simulink library "BodyLoad_Tank_Cylindrical"  (R2025b)
settings: Solver=VariableStepAuto  StartTime=0.0  StopTime=10.0  RelTol=1e-3
undefined symbols (not defined in the file): BodyLoad, X, Y, Z
libraries: sm_lib x4
Description:
  | Component of Simscape Vehicle Templates Library
  | 
  | Copyright 2018-2025 The MathWorks, Inc.
settings Model: Creator=smiller  LastModifiedBy=smiller
settings SolverCC: AlgebraicLoopSolver=TrustRegion
settings DataIOCC: ReturnWorkspaceOutputs=off
settings OptimizationCC: ReuseModelBlockBuffer=off
settings DebuggingCC: UnconnectedInputMsg=warning  UnconnectedOutputMsg=warning  UnconnectedLineMsg=warning  ArithmeticOperatorsInVariantConditions=warning
settings ModelReferenceCC: EnableRefExpFcnMdlSchedulingChecks=on
settings SFSimCC: CustomCodeUndefinedFunction=UseInterfaceOnly
settings RTWCC: GPUComputeCapability=3.5  DLArmComputeVersion=19.05

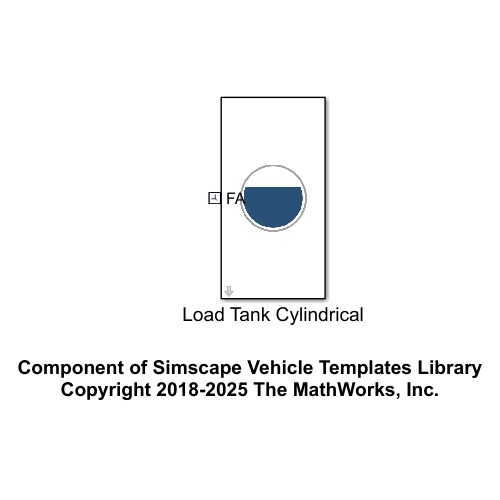
[thumbnail: Simulink's stored preview of the top-level diagram]
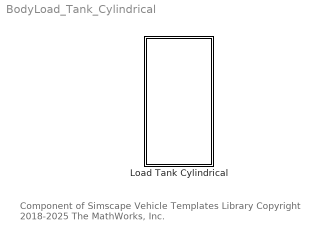
== system BodyLoad_Tank_Cylindrical ==
  note: Component of Simscape Vehicle Templates Library
      | Copyright 2018-2025 The MathWorks, Inc.
  Load Tank Cylindrical : Subsystem  mask(Inertial Load for Cylindrical Tank){refToTankCtr=BodyLoad.xRefToTankCtr.Value, tank_rad=BodyLoad.xRadius.Value, tank_len=BodyLoad.xLength.Value, pcnt_fill=BodyLoad.rFillHeight.Value, rho=BodyLoad.rho.Value, dLoad=BodyLoad.dLoad.Value, clr=BodyLoad.Color.Value, opc=BodyLoad.Opacity.Value}
      mask prompts: refToTankCtr "Ref to Tank Center [x y z] (m)"; tank_rad "Tank Radius (m)"; tank_len "Tank Length (m)"; pcnt_fill "Percent Fill Height (0-1)"; rho "Density (kg/m^3)"; dLoad "Load Rotational Damping (N*m/(deg/s))"; clr "Color [RGB]"; opc "Opacity (0-1)"
      mask help: Model the load in a full or partially full horizontal cylindrical tank subjected to gravity. Specify the size of the tank, density of the fluid, and how full the tank is. Tank fill level is specified as a percentage of the tank diameter. The load can slosh laterally by rotating around the tank axis. Slosh can be inibited by setting the Load Rotational Damping to a high value.
      mask init:
      | % Limit percent fill from 0-1
      | if(pcnt_fill>1)
      |     pcnt_fill = 1;
      | elseif(pcnt_fill<0)
      |     pcnt_fill = 0;
      | end
      | 
      | % Calculate angle for extrusion
      | if(pcnt_fill>0.5)
      |     fill_angle = pi/2+asin((pcnt_fill-0.5)*2);
      | else
      |     fill_angle = acos((0.5-pcnt_fill)*2);
      | end
      | 
      | % Create angle vector for extrusion
      | angle_vec = linspace(-fill_angle,fill_angle,50);
      | 
      | % Create extrusion data
      | xy_data_load = [(cos(angle_vec))' (sin(angle_vec))']*(tank_rad-1e-3);
      mask TypeOptions clr: Load/GraphicDiffuseColor
      mask TypeOptions opc: Load/GraphicOpacity
      mask DialogControl cont_vis Prompt: Visualization
      mask Display: image('sm_car_vehicle_bodyload_slosh_tankcyl_IMAGE.png');

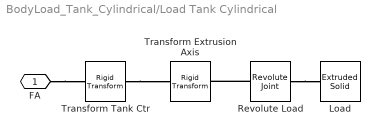
== system BodyLoad_Tank_Cylindrical/Load Tank Cylindrical ==
  Load : sm_lib/Body Elements/Extruded Solid  ExtrusionType=General  PolygonNumSides=3  PolygonOuterRadius=1  PolygonOuterRadiusUnits=m  ExportEntireGeometry=off  ExtrusionCrossSection=xy_data_load  ExtrusionCrossSectionUnits=m  ExportConvexHullGeometry=off  ExtrusionLength=tank_len  ExtrusionLengthUnits=m  InertiaType=CalculateFromGeometry  BasedOnType=Density  Density=rho  DensityUnits=kg/m^3  Mass=1  MassUnits=kg  CenterOfMass=[0 0 0]  CenterOfMassUnits=m  MomentsOfInertia=[1 1 1]  MomentsOfInertiaUnits=kg*m^2  ProductsOfInertia=[0 0 0]  ProductsOfInertiaUnits=kg*m^2  GraphicType=FromGeometry  MarkerShape=Sphere  MarkerSize=10  GraphicVisPropType=SimpleVisualProperties  GraphicDiffuseColor=clr  GraphicOpacity=opc  GraphicSpecularColor=[0.5 0.5 0.5 1.0]  GraphicAmbientColor=[0.15 0.15 0.15 1.0]  GraphicEmissiveColor=[0.0 0.0 0.0 1.0]  GraphicShininess=75  DoExposeReferenceFrame=on  SerializedFrames=<Frames/>
  Revolute Load : sm_lib/Joints/Revolute Joint  JointMode=Normal  CompositeWrenchDir=FollowerOnBase  CompositeWrenchFrame=BaseFrame  SenseConstraintForce=off  SenseConstraintTorque=off  SenseTotalForce=off  SenseTotalTorque=off  PositionTargetSpecify=off  PositionTargetPriority=High  PositionTargetValue=0  PositionTargetValueUnits=deg  VelocityTargetSpecify=off  VelocityTargetPriority=High  VelocityTargetValue=0  VelocityTargetValueUnits=deg/s  EquilibriumPosition=0  EquilibriumPositionUnits=deg  SpringStiffness=0  SpringStiffnessUnits=N*m/deg  DampingCoefficient=dLoad  DampingCoefficientUnits=N*m/(deg/s)  LowerLimitSpecify=off  LowerLimitBound=-90  LowerLimitBoundUnits=deg  LowerLimitStiffness=1e4  LowerLimitStiffnessUnits=N*m/deg  LowerLimitDamping=10  LowerLimitDampingUnits=N*m/(deg/s)  LowerLimitTransitionRegionWidth=0.1  LowerLimitTransitionRegionWidthUnits=deg  UpperLimitSpecify=off  UpperLimitBound=90  UpperLimitBoundUnits=deg  UpperLimitStiffness=1e4  UpperLimitStiffnessUnits=N*m/deg  UpperLimitDamping=10  UpperLimitDampingUnits=N*m/(deg/s)  UpperLimitTransitionRegionWidth=0.1  UpperLimitTransitionRegionWidthUnits=deg  TorqueActuationMode=NoTorque  MotionActuationMode=ComputedMotion  SensePosition=off  SenseVelocity=off  SenseAcceleration=off  SenseTorqueForce=off  SenseLowerLimitTorqueForce=off  SenseUpperLimitTorqueForce=off
  Transform Extrusion Axis : sm_lib/Frames and Transforms/Rigid Transform  RotationMethod=StandardAxis  FollAlignAxisA=+X  BaseAlignAxisA=+Y  FollAlignAxisB=+Y  BaseAlignAxisB=+Z  RotationStandardAxis=+Y  RotationAngle=90  RotationAngleUnits=deg  RotationArbitraryAxis=[0 0 1]  RotationSequenceAxes=FollowerAxes  RotationSequence=XYX  RotationSequenceAngles=[0 0 0]  RotationSequenceAnglesUnits=deg  RotationMatrix=[1 0 0; 0 1 0; 0 0 1]  Quaternion=[1 0 0 0]  TranslationMethod=None  TranslationCartesianOffset=[0 0 0]  TranslationCartesianOffsetUnits=m  TranslationStandardAxis=+Z  TranslationStandardOffset=0  TranslationStandardOffsetUnits=m  TranslationROffset=0  TranslationROffsetUnits=m  TranslationThetaOffset=0  TranslationThetaOffsetUnits=deg  TranslationZOffset=0  TranslationZOffsetUnits=m
  Transform Tank Ctr : sm_lib/Frames and Transforms/Rigid Transform  RotationMethod=None  FollAlignAxisA=+X  BaseAlignAxisA=+Y  FollAlignAxisB=+Y  BaseAlignAxisB=+Z  RotationStandardAxis=+Z  RotationAngle=0.0  RotationAngleUnits=deg  RotationArbitraryAxis=[0 0 1]  RotationSequenceAxes=FollowerAxes  RotationSequence=XYX  RotationSequenceAngles=[0 0 0]  RotationSequenceAnglesUnits=deg  RotationMatrix=[1 0 0; 0 1 0; 0 0 1]  Quaternion=[1 0 0 0]  TranslationMethod=Cartesian  TranslationCartesianOffset=refToTankCtr  TranslationCartesianOffsetUnits=m  TranslationStandardAxis=+Z  TranslationStandardOffset=0  TranslationStandardOffsetUnits=m  TranslationROffset=0  TranslationROffsetUnits=m  TranslationThetaOffset=0  TranslationThetaOffsetUnits=deg  TranslationZOffset=0  TranslationZOffsetUnits=m
  FA : PMIOPort  Side=Left
  connections:
  Transform Tank Ctr/RConn1 -- Transform Extrusion Axis/LConn1
  FA/RConn1 -- Transform Tank Ctr/LConn1
  Revolute Load/LConn1 -- Transform Extrusion Axis/RConn1
  Revolute Load/RConn1 -- Load/RConn1
